simulink model "ReqsGroundTruth_Harness2"  (R2021b)
settings: Solver=FixedStepAuto  StartTime=0.0  StopTime=stopTime  RelTol=1e-3
settings Model: Creator=akshran  LastModifiedBy=akshran
settings OptimizationCC: DefaultParameterBehavior=Inlined  EnhancedBackFolding=on  PassReuseOutputArgsAs=Individual arguments  ZeroExternalMemoryAtStartup=off  ZeroInternalMemoryAtStartup=off  OptimizeBlockOrder=speed  DifferentSizesBufferReuse=on  OptimizationCustomize=off  EfficientTunableParamExpr=on
settings DebuggingCC: ParameterTunabilityLossMsg=error
settings SFSimCC: MATLABDynamicMemAlloc=off
settings RTWCC: Description=Embedded Coder  SystemTargetFile=ert.tlc  TemplateMakefile=ert_default_tmf  BuildConfiguration=Faster Runs  CodeExecutionProfiling=on  CodeProfilingSaveOptions=AllData  TargetLang=C++
settings CodeAppCC: ForceParamTrailComments=on  IgnoreCustomStorageClasses=off  OperatorAnnotations=on  SimulinkDataObjDesc=on  SFDataObjDesc=on  InsertBlockDesc=on
settings ERTTargetCC: TargetLangStandard=C++11 (ISO)  GenerateSampleERTMain=on  CodeInterfacePackaging=C++ class  SupportContinuousTime=on  SupportVariableSizeSignals=on  InlinedParameterPlacement=NonHierarchical  RootIOFormat=Structure reference  ERTCustomFileTemplate=example_file_process.tlc
settings ConfigComp: CovEnable=on  CovScope=ReferencedModels  CovIncludeTopModel=off  CovMetricSettings=dtrzoibwe  CovModelRefEnable=filtered

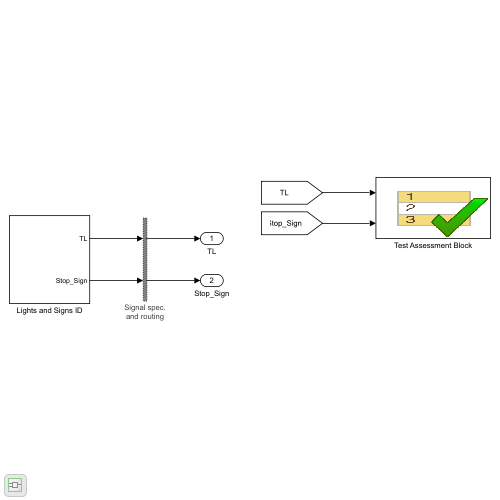
[thumbnail: Simulink's stored preview of the top-level diagram]
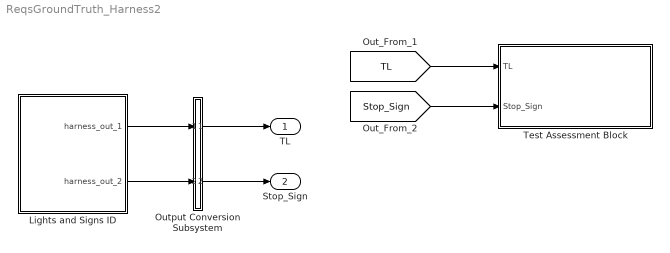
== system ReqsGroundTruth_Harness2 ==
  Lights and Signs ID : Subsystem  Tag=__SL_testing_harness_stub_
  Output Conversion Subsystem : Subsystem  Tag=__SLT_OCS__  Description=|
      | Signal spec.
      | and routing
      settings: AttributesFormatString=%<Description>
  Test Assessment Block : Test Sequence  Tag=__SLT_ASMT__  TreatAsAtomicUnit=on
  TL : Outport
  Stop_Sign : Outport  Port=2
  wires:
  [TL] -> Test Assessment Block/1(TL)
  [Stop_Sign] -> Test Assessment Block/2(Stop_Sign)
  Output Conversion Subsystem/1(Outport_1) -> TL/1
  Output Conversion Subsystem/2(Outport_2) -> Stop_Sign/1
  Lights and Signs ID/1(harness_out_1) -> Output Conversion Subsystem/1(Inport_1)
  Lights and Signs ID/2(harness_out_2) -> Output Conversion Subsystem/2(Inport_2)

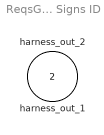
== system ReqsGroundTruth_Harness2/Lights and Signs ID ==
  harness_out_1 : Outport
  harness_out_2 : Outport  Port=2

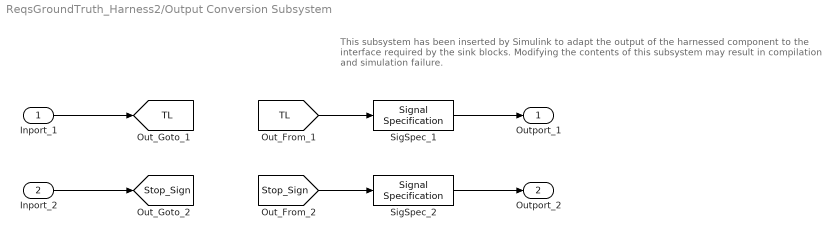
== system ReqsGroundTruth_Harness2/Output Conversion Subsystem ==
  note: This subsystem has been inserted by Simulink to adapt the output of the harnessed component to the interface required by the sink blocks.
      |  Modifying the contents of this subsystem may result in compilation and simulation failure.
  Inport_1 : Inport
  Inport_2 : Inport  Port=2
  SigSpec_1 : SignalSpecification  OutDataTypeStr=double  Dimensions=[1]
  SigSpec_2 : SignalSpecification  OutDataTypeStr=double  Dimensions=[1]
  Outport_1 : Outport
  Outport_2 : Outport  Port=2
  tag scope: Stop_Sign=global, TL=global
  wires:
  Inport_1/1 -> [TL]
  [TL] -> SigSpec_1/1
  SigSpec_1/1 -> Outport_1/1
  Inport_2/1 -> [Stop_Sign]
  [Stop_Sign] -> SigSpec_2/1
  SigSpec_2/1 -> Outport_2/1

== stateflow chart ReqsGroundTruth_Harness2/Test Assessment Block ==
  state Assessments
    state VerifyThis
      verify(numel(TL)==2,'Scenario Contains req traffic lights')
      verify(numel(Stop_Sign)==1,'Scenario Contains req stop signs')
    state End
    (default) -> (junction 22)
    Assessments -> (junction 22)
    (junction 22) -> (junction 23) [order 1] : [t==0
        | ]
    (junction 23) -> VerifyThis [order 1] : [~in(Assessments.VerifyThis)]
    (junction 22) -> (junction 31) [order 2]
    (junction 23) -> (junction 26) [order 2]
    (junction 31) -> (junction 32)
    (junction 32) -> End [order 1] : [~in(Assessments.End)]
    (junction 32) -> (junction 35) [order 2]
  (default) -> Assessments
  data: TL input double size=[1]; Stop_Sign input double size=[1]
